simulink model "calibration"  (R2018a)
settings: Solver=VariableStepAuto  StartTime=0.0  StopTime=60  RelTol=1e-3
values from neighbouring files (symbols this model uses):
  brake = brake+0.1    (= 0.2)    [brake_calibration.m]
  thr = thr+0.01    (= 0.01)    [thr_calibration.m]
libraries: Solver_SF x1
settings Model: Creator=wwcong  LastModifiedBy=wwcong

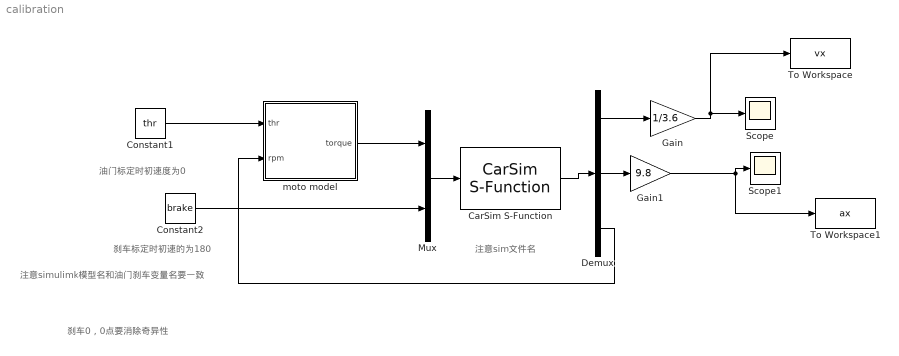
== system calibration ==
  note: 刹车0，0点要消除奇异性
  note: 注意simulimk模型名和油门刹车变量名要一致
  note: 刹车标定时初速的为180
  note: 油门标定时初速度为0
  note: 注意sim文件名
  CarSim S-Function : Solver_SF/CarSim S-Function  Priority=1  VehicleCode=i_i  SIMFILE=calibration.sim
  Constant1 : Constant  Value=thr
  Constant2 : Constant  Value=brake
  Demux : Demux  Outputs=3
  Gain : Gain  Gain=1/3.6
  Gain1 : Gain  Gain=9.8
  Mux : Mux  Inputs=2
  Scope : Scope
  Scope1 : Scope
  To Workspace : ToWorkspace  VariableName=vx  SaveFormat=Timeseries  SampleTime=0.1
  To Workspace1 : ToWorkspace  VariableName=ax  SaveFormat=Timeseries  SampleTime=0.1
  moto model : MATLAB Function  TreatAsAtomicUnit=on
  wires:
  Mux/1 -> CarSim S-Function/1
  CarSim S-Function/1 -> Demux/1
  Demux/1 -> Gain/1
  Demux/2 -> Gain1/1
  Gain1/1 -> To Workspace1/1, Scope1/1
  Gain/1 -> To Workspace/1, Scope/1
  Demux/3 -> moto model/2(rpm)
  moto model/1(torque) -> Mux/1
  Constant1/1 -> moto model/1(thr)
  Constant2/1 -> Mux/2

== matlab function calibration/moto model ==
  data: thr input; torque output; rpm input
function torque = fcn(thr,rpm)
Tmax=380*thr;
    if (rpm<=4523)
        torque=Tmax;
    else
        torque=Tmax*4523/rpm;
    end
end
